simulink model "comparative_study"  (R2025b)
settings: Solver=ode4  StartTime=0.0  StopTime=15  FixedStep=0.01  RelTol=1e-3
model workspace (MAT data in the model file):
  L = 2.65
  Lh = 0
  k = 1
  theta_d = 1
values from neighbouring files (symbols this model uses):
  K = dlqr(Ad, Bd, Q, R)    [lqr_hw.m]
  K_mpc = K_full(1, :)    [mpc_hw.m]
settings Model: Creator=yasin  LastModifiedBy=yasin

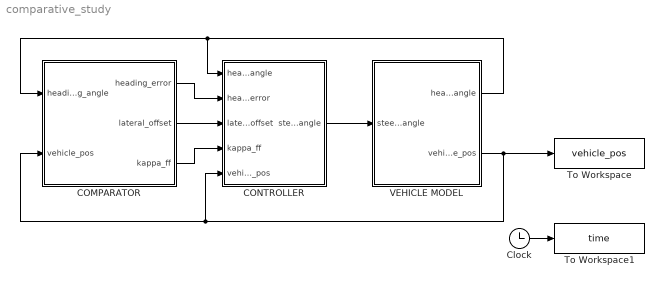
== system comparative_study ==
  COMPARATOR : Subsystem
  CONTROLLER : Subsystem
  Clock : Clock
  To Workspace : ToWorkspace  VariableName=vehicle_pos  SampleTime=-1
  To Workspace1 : ToWorkspace  VariableName=time  SampleTime=-1
  VEHICLE MODEL : Subsystem
  wires:
  COMPARATOR/1(heading_error) -> CONTROLLER/2(heading_error)
  COMPARATOR/2(lateral_offset) -> CONTROLLER/3(lateral_offset)
  VEHICLE MODEL/1(heading_angle) -> CONTROLLER/1(heading_angle), COMPARATOR/1(heading_angle)
  VEHICLE MODEL/2(vehicle_pos) -> To Workspace/1, CONTROLLER/5(vehicle_pos), COMPARATOR/2(vehicle_pos)
  Clock/1 -> To Workspace1/1
  CONTROLLER/1(steering_angle) -> VEHICLE MODEL/1(steering_angle)
  COMPARATOR/3(kappa_ff) -> CONTROLLER/4(kappa_ff)

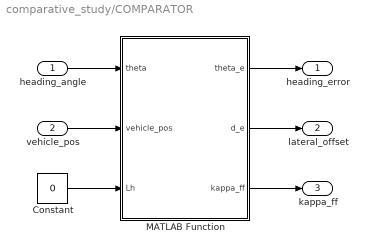
== system comparative_study/COMPARATOR ==
  heading_angle : Inport
  vehicle_pos : Inport  Port=2
  Constant : Constant  Value=0
  MATLAB Function : MATLAB Function  TreatAsAtomicUnit=on
  heading_error : Outport
  lateral_offset : Outport  Port=2
  kappa_ff : Outport  Port=3
  wires:
  heading_angle/1 -> MATLAB Function/1(theta)
  vehicle_pos/1 -> MATLAB Function/2(vehicle_pos)
  MATLAB Function/1(theta_e) -> heading_error/1
  MATLAB Function/2(d_e) -> lateral_offset/1
  Constant/1 -> MATLAB Function/3(Lh)
  MATLAB Function/3(kappa_ff) -> kappa_ff/1

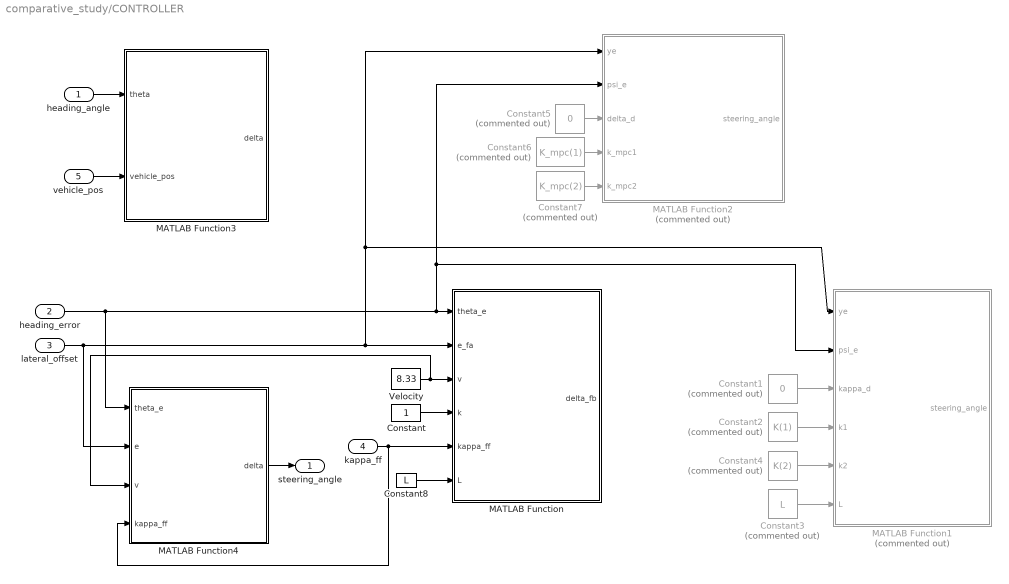
== system comparative_study/CONTROLLER ==
  heading_angle : Inport
  heading_error : Inport  Port=2
  lateral_offset : Inport  Port=3
  kappa_ff : Inport  Port=4
  vehicle_pos : Inport  Port=5
  Constant : Constant
  Constant1 : Constant  Commented=on  Value=0
  Constant2 : Constant  Commented=on  Value=K(1)
  Constant3 : Constant  Commented=on  Value=L
  Constant4 : Constant  Commented=on  Value=K(2)
  Constant5 : Constant  Commented=on  Value=0
  Constant6 : Constant  Commented=on  Value=K_mpc(1)
  Constant7 : Constant  Commented=on  Value=K_mpc(2)
  Constant8 : Constant  Value=L
  MATLAB Function : MATLAB Function  TreatAsAtomicUnit=on
  MATLAB Function1 : MATLAB Function  Commented=on  TreatAsAtomicUnit=on
  MATLAB Function2 : MATLAB Function  Commented=on  TreatAsAtomicUnit=on
  MATLAB Function3 : MATLAB Function  TreatAsAtomicUnit=on
  MATLAB Function4 : MATLAB Function  TreatAsAtomicUnit=on
  Velocity : Constant  Value=8.33
  steering_angle : Outport
  wires:
  heading_error/1 -> MATLAB Function4/1(theta_e), MATLAB Function1/2(psi_e), MATLAB Function2/2(psi_e), MATLAB Function/1(theta_e)
  lateral_offset/1 -> MATLAB Function4/2(e), MATLAB Function/2(e_fa), MATLAB Function1/1(ye), MATLAB Function2/1(ye)
  Velocity/1 -> MATLAB Function4/3(v), MATLAB Function/3(v)
  Constant/1 -> MATLAB Function/4(k)
  Constant1/1 -> MATLAB Function1/3(kappa_d)
  Constant2/1 -> MATLAB Function1/4(k1)
  Constant3/1 -> MATLAB Function1/6(L)
  Constant4/1 -> MATLAB Function1/5(k2)
  Constant5/1 -> MATLAB Function2/3(delta_d)
  Constant6/1 -> MATLAB Function2/4(k_mpc1)
  Constant7/1 -> MATLAB Function2/5(k_mpc2)
  kappa_ff/1 -> MATLAB Function4/4(kappa_ff), MATLAB Function/5(kappa_ff)
  Constant8/1 -> MATLAB Function/6(L)
  vehicle_pos/1 -> MATLAB Function3/2(vehicle_pos)
  heading_angle/1 -> MATLAB Function3/1(theta)
  MATLAB Function4/1(delta) -> steering_angle/1

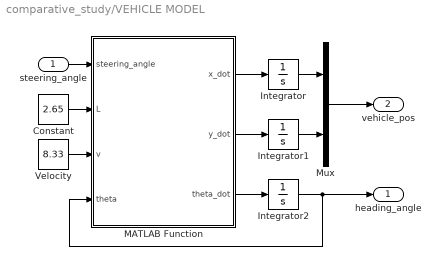
== system comparative_study/VEHICLE MODEL ==
  steering_angle : Inport
  Constant : Constant  Value=2.65
  Integrator : Integrator
  Integrator1 : Integrator
  Integrator2 : Integrator
  MATLAB Function : MATLAB Function  TreatAsAtomicUnit=on
  Mux : Mux  Inputs=2
  Velocity : Constant  Value=8.33
  heading_angle : Outport
  vehicle_pos : Outport  Port=2
  wires:
  steering_angle/1 -> MATLAB Function/1(steering_angle)
  Constant/1 -> MATLAB Function/2(L)
  MATLAB Function/1(x_dot) -> Integrator/1
  MATLAB Function/2(y_dot) -> Integrator1/1
  MATLAB Function/3(theta_dot) -> Integrator2/1
  Mux/1 -> vehicle_pos/1
  Integrator2/1 -> MATLAB Function/4(theta), heading_angle/1
  Integrator/1 -> Mux/1
  Integrator1/1 -> Mux/2
  Velocity/1 -> MATLAB Function/3(v)

== matlab function comparative_study/COMPARATOR/MATLAB Function ==
  data: theta input; theta_e output; vehicle_pos input; d_e output; Lh input; kappa_ff output
function [theta_e, d_e, kappa_ff] = fcn(theta, vehicle_pos, Lh)

x = vehicle_pos(1);
y = vehicle_pos(2);

% --- Referans yol: düz çizgi + sol yay (curvature'ı olan bir yol) ---
ds  = 0.1;
xs1 = 0:ds:50;               y1 = zeros(1, numel(xs1));     % düz
R   = 20;  th = ds/R : ds/R : pi/2;                          % yay (th=0 atlandı)
x2  = 50 + R*sin(th);        y2 = R - R*cos(th);
x_d = [xs1, x2];             y_d = [y1, y2];

% --- enhancement parametreleri (CONTROLLER'daki Velocity ile eşleşmeli) ---
v    = 8;        % m/s
t_ff = 0.18;     % s  (makale: sim 0.18 / araç 0.20)

% --- yay uzunluğu, teğet açısı, işaretli curvature ---
seg     = hypot(diff(x_d), diff(y_d));
s_d     = [0, cumsum(seg)];
dx = gradient(x_d);   dy = gradient(y_d);
ddx = gradient(dx);   ddy = gradient(dy);
psi_d   = atan2(dy, dx);
kappa_d = (dx.*ddy - dy.*ddx) ./ ((dx.^2 + dy.^2).^1.5 + 1e-9);

% --- en yakın nokta ---
[~, idx] = min((x - x_d).^2 + (y - y_d).^2);
theta_d  = psi_d(idx);
theta_e  = theta_d - theta;

x_near = x_d(idx);  y_near = y_d(idx);
d_e = (x + Lh*cos(theta) - x_near)*sin(theta_d) ...
    + (-y - Lh*sin(theta) + y_near)*cos(theta_d);

% --- ENHANCEMENT: lookahead noktasındaki curvature  (s_ff = v*t_ff) ---
s_look   = s_d(idx) + v*t_ff;
s_look   = min(max(s_look, s_d(1)), s_d(end));
kappa_ff = interp1(s_d, kappa_d, s_look, 'linear');

== matlab function comparative_study/VEHICLE MODEL/MATLAB Function ==
  data: steering_angle input; x_dot output; y_dot output; L input; v input; theta_dot output; theta input
function [x_dot, y_dot, theta_dot]  = fcn(steering_angle, L, v, theta)

x_dot     = v*cos(theta);
y_dot     = v*sin(theta);
theta_dot = v*tan(steering_angle)/L;

== matlab function comparative_study/CONTROLLER/MATLAB Function ==
  data: theta_e input; delta_fb output; e_fa input; v input; k input; kappa_ff input; L input
function delta_fb = stanley(theta_e, e_fa, v, k, kappa_ff, L)

delta_ff = atan(L * kappa_ff);
delta_fb = theta_e + atan(k*e_fa / v);
steering_angle = delta_ff + delta_fb;

== matlab function comparative_study/CONTROLLER/MATLAB Function1 ==
  data: ye input; steering_angle output; psi_e input; kappa_d input; k1 input; k2 input; L input
function steering_angle = lqr_steer(ye, psi_e, kappa_d, k1, k2, L)

u_fb = (k1*ye + k2*psi_e);
steering_angle_ff = atan(L * kappa_d);
steering_angle = u_fb + steering_angle_ff;

steering_angle_max = deg2rad(35);
if steering_angle >  steering_angle_max,  steering_angle =  steering_angle_max; end
if steering_angle < -steering_angle_max,  steering_angle = -steering_angle_max; end

== matlab function comparative_study/CONTROLLER/MATLAB Function2 ==
  data: ye input; steering_angle output; psi_e input; delta_d input; k_mpc1 input; k_mpc2 input
function steering_angle = mpc_controller(ye, psi_e, delta_d, k_mpc1, k_mpc2)

du = k_mpc1*ye + k_mpc2*psi_e;
steering_angle = delta_d + du;

== matlab function comparative_study/CONTROLLER/MATLAB Function3 ==
  data: theta input; delta output; vehicle_pos input
function delta = predictive_stanley(theta, vehicle_pos)
% Mevcut poz + N tahmini pozda basic Stanley'in ağırlıklı toplamı.
% Harici Memory/feedback YOK. Girişler: theta, vehicle_pos. Çıkış: delta.

% --- ayarlar ---
v   = 8.33;            % Velocity ile aynı tut
k   = 1;            % basic Stanley kazancı ile aynı
L   = 2.65;  Lh = L;
K0  = 0.95;         % mevcut poz ağırlığı
KfT = 0.05;         % toplam gelecek ağırlığı (K0+KfT = 1)
N   = 5;            % tahmin adımı sayısı
dlt = 0.3;          % tahmin zaman adımı Δ (s)

% --- path (comparator ile birebir aynı) ---
ds = 0.1;
xs1 = 0:ds:50;          y1 = zeros(1, numel(xs1));
R = 20;  th = ds/R:ds/R:pi/2;
x2 = 50 + R*sin(th);    y2 = R - R*cos(th);
x_d = [xs1, x2];        y_d = [y1, y2];
dx = gradient(x_d);  dy = gradient(y_d);
psi_d = atan2(dy, dx);

x = vehicle_pos(1);  y = vehicle_pos(2);

% --- mevcut poz: basic Stanley ---
[~, i0] = min((x - x_d).^2 + (y - y_d).^2);
td = psi_d(i0);
e  = (x + Lh*cos(theta) - x_d(i0))*sin(td) + (-y - Lh*sin(theta) + y_d(i0))*cos(td);
d0 = (td - theta) + atan(k*e/v);
delta = K0 * d0;

% --- N adım ileri tahmin (d0 sabit, plant kinematiğiyle aynı) ---
Kf = KfT / N;
xp = x;  yp = y;  thp = theta;
for n = 1:N
    xp  = xp + v*cos(thp)*dlt;
    yp  = yp + v*sin(thp)*dlt;
    thp = thp + (v*tan(d0)/L)*dlt;
    [~, ip] = min((xp - x_d).^2 + (yp - y_d).^2);
    tdp = psi_d(ip);
    ep  = (xp + Lh*cos(thp) - x_d(ip))*sin(tdp) + (-yp - Lh*sin(thp) + y_d(ip))*cos(tdp);
    delta = delta + Kf*((tdp - thp) + atan(k*ep/v));
end

== matlab function comparative_study/CONTROLLER/MATLAB Function4 ==
  data: theta_e input; delta output; e input; v input; kappa_ff input
function delta = adaptive_stanley(theta_e, e, v, kappa_ff)
tp_max = 0.2;        % düz yolda preview time (1/k_basic seç -> düzde basic'le çakışsın)
tp_min = 0.08;       % keskin virajda preview time
kref   = 0.05;       % normalizasyon eğriliği (1/R = 1/20)

w  = min(abs(kappa_ff)/kref, 1);
tp = tp_max - (tp_max - tp_min)*w;
delta = theta_e + atan(e / (tp * v));
end
